simulink model "parrot_vision"  (R2020b)
settings: Solver=FixedStepAuto  StartTime=0.0  StopTime=100  RelTol=1e-3  EnableMultiTasking=on
InitFcn:
  | load('BusDefinitions.mat')
  | codertarget.parrot.internal.checkImageBlocks(gcs)
undefined symbols (not defined in the file): codertarget, Ts
libraries: simulink x3, parrotlib x1
settings Model: ExtModeTrigDuration=80  Creator=The MathWorks, Inc.  LastModifiedBy=anne
settings SolverCC: PositivePriorityOrder=on
settings DataIOCC: ReturnWorkspaceOutputs=off
settings OptimizationCC: PassReuseOutputArgsThreshold=0  MaxStackSize=64
settings DebuggingCC: ParameterTunabilityLossMsg=error  PregeneratedLibrarySubsystemCodeDiagnostic=none  ArithmeticOperatorsInVariantConditions=warning
settings HardwareCC: ProdBitPerPointer=32  ProdBitPerSizeT=32  ProdBitPerPtrDiffT=32  ProdLargestAtomicInteger=Long  ProdWordSize=32  ProdHWDeviceType=ARM Compatible->ARM 9  UseEmbeddedCoderFeatures=off  UseSimulinkCoderFeatures=off
settings SFSimCC: SimUseLocalCustomCode=off  MATLABDynamicMemAlloc=off  CustomCodeUndefinedFunction=UseInterfaceOnly
settings RTWCC: Description=Embedded Coder  SystemTargetFile=ert.tlc  HardwareBoard=PARROT Mambo  TemplateMakefile=ert_default_tmf  GenerateReport=on  RTWUseLocalCustomCode=off  Toolchain=Sourcery G++ Lite GNU Toolchain for Drones  LaunchReport=on
settings CodeAppCC: ForceParamTrailComments=on  OperatorAnnotations=on  StateflowObjectComments=on
settings ERTTargetCC: ERTCustomFileBanners=off  SupportContinuousTime=on  SupportNonInlinedSFcns=on  RemoveResetFunc=off  ModelStepFunctionPrototypeControlCompliant=off

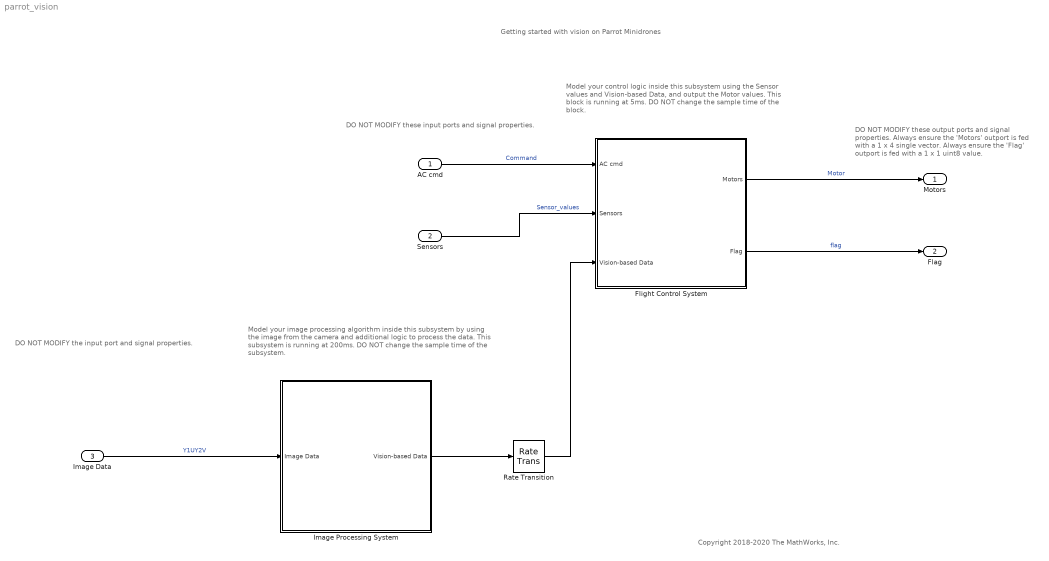
== system parrot_vision ==
  note: Model your control logic inside this subsystem
      | using the Sensor values and Vision-based Data,
      | and output the Motor values.
      | This block is running at 5ms.
      | DO NOT change the sample time of the block.
  note: DO NOT MODIFY these output ports
      | and signal properties.
      |
      |
      |
      |
      |
      | Always ensure the 'Motors' outport
      | is fed with a 1 x 4 single vector.
      |
      |
      |
      |
      |
      | Always ensure the 'Flag' outport is
      | fed with a 1 x 1 uint8 value.
  note: DO NOT MODIFY these input
      | ports and signal properties.
  note: Copyright 2018-2020 The MathWorks, Inc.
  note: Getting started with vision on Parrot Minidrones
  note: DO NOT MODIFY the input port and
      | signal properties.
  note: Model your image processing algorithm inside this
      | subsystem by using the image from the camera
      | and additional logic to process the data.
      | This subsystem is running at 200ms.
      | DO NOT change the sample time of the subsystem.
  AC cmd : Inport  OutDataTypeStr=Bus: CommandBus  BusOutputAsStruct=on
  Sensors : Inport  Port=2  OutDataTypeStr=Bus: SensorsBus  BusOutputAsStruct=on
  Image Data : Inport  Tag=IP_IN  InitFcn=codertarget.parrot.internal.inportCallback(gcb);  Port=3  OutDataTypeStr=uint8  PortDimensions=[4 9600]  BusOutputAsStruct=on
  Flight Control System : Subsystem  InitFcn=codertarget.parrot.internal.fcsSubsystemCallback(gcb);  TreatAsAtomicUnit=on  SystemSampleTime=Ts
  Image Processing System : Subsystem  Tag=IP_SUB  InitFcn=codertarget.parrot.internal.ipSubsystemCallback(gcb);  TreatAsAtomicUnit=on  SystemSampleTime=40*Ts  RTWFcnName=ImageFunction
      settings: RTWSystemCode=Inline  RTWFcnNameOpts=User specified
  Rate Transition : RateTransition  Deterministic=off
  Motors : Outport  OutDataTypeStr=single  PortDimensions=[1 4]  VectorParamsAs1DForOutWhenUnconnected=off
  Flag : Outport  Port=2  OutDataTypeStr=uint8  PortDimensions=1  VectorParamsAs1DForOutWhenUnconnected=off
  wires:
  Flight Control System/1(Motors) -> Motors/1  "Motor"
  AC cmd/1 -> Flight Control System/1(AC cmd)  "Command"
  Sensors/1 -> Flight Control System/2(Sensors)  "Sensor_values"
  Flight Control System/2(Flag) -> Flag/1  "flag"
  Image Data/1 -> Image Processing System/1(Image Data)  "Y1UY2V"
  Rate Transition/1 -> Flight Control System/3(" Vision-based Data")
  Image Processing System/1(" Vision-based Data") -> Rate Transition/1

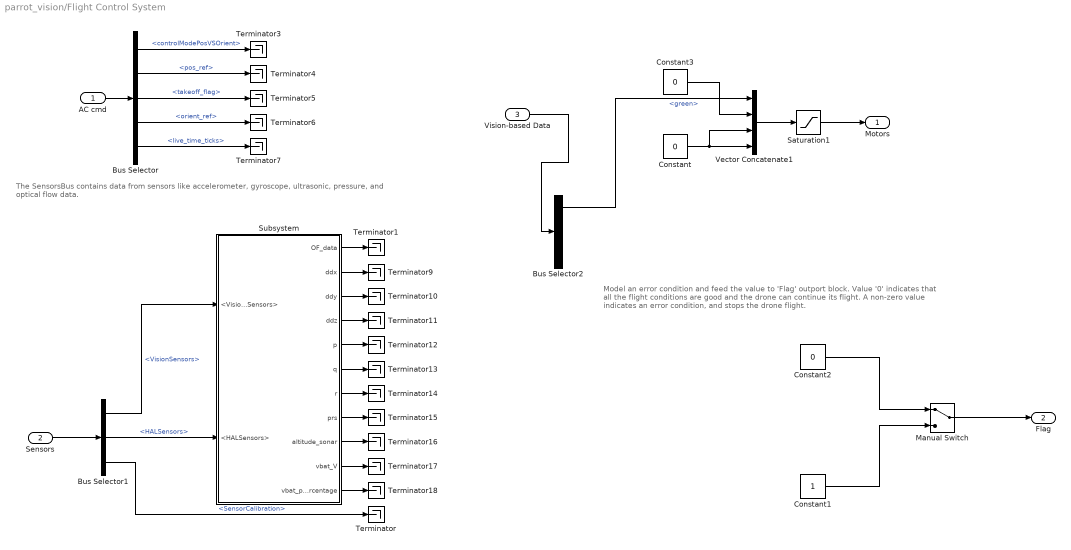
== system parrot_vision/Flight Control System ==
  note: Model an error condition and feed the value to 'Flag' outport block.
      | Value '0' indicates that all the flight conditions are good and the drone
      | can continue its flight.
      | A non-zero value indicates an error condition, and stops the drone
      | flight.
  note: The SensorsBus contains data from sensors like
      | accelerometer, gyroscope, ultrasonic, pressure,
      | and optical flow data.
  AC cmd : Inport
  Sensors : Inport  Port=2
  " Vision-based Data" : Inport  Port=3
  Bus Selector : BusSelector  OutputSignals=controlModePosVSOrient,pos_ref,takeoff_flag,orient_ref,live_time_ticks
  Bus Selector1 : BusSelector  OutputSignals=VisionSensors,HALSensors,SensorCalibration
  Bus Selector2 : BusSelector  OutputSignals=green,red,blue
  Constant : Constant  Value=0
  Constant1 : Constant  OutDataTypeStr=uint8
  Constant2 : Constant  Value=0  OutDataTypeStr=uint8
  Constant3 : Constant  Value=0
  Manual Switch : ManualSwitch
  Saturation1 : Saturate  UpperLimit=500  LowerLimit=0  OutDataTypeStr=single
  Subsystem : Subsystem
  Terminator{,1,3..7,9..18} (17 alike) : Terminator
  Vector Concatenate1 : Concatenate  NumInputs=4
  Motors : Outport  VectorParamsAs1DForOutWhenUnconnected=off
  Flag : Outport  Port=2  VectorParamsAs1DForOutWhenUnconnected=off
  wires:
  AC cmd/1 -> Bus Selector/1
  Sensors/1 -> Bus Selector1/1
  Bus Selector/1 -> Terminator3/1  "<controlModePosVSOrient>"
  Bus Selector/2 -> Terminator4/1  "<pos_ref>"
  Bus Selector/3 -> Terminator5/1  "<takeoff_flag>"
  Bus Selector/4 -> Terminator6/1  "<orient_ref>"
  Bus Selector/5 -> Terminator7/1  "<live_time_ticks>"
  Manual Switch/1 -> Flag/1
  Constant2/1 -> Manual Switch/1
  Constant1/1 -> Manual Switch/2
  Vector Concatenate1/1 -> Saturation1/1
  Saturation1/1 -> Motors/1
  Bus Selector1/1 -> Subsystem/1(<VisionSensors>)  "<VisionSensors>"
  Bus Selector1/2 -> Subsystem/2(<HALSensors>)  "<HALSensors>"
  Bus Selector1/3 -> Terminator/1  "<SensorCalibration>"
  Subsystem/1(OF_data) -> Terminator1/1
  Subsystem/2(ddx) -> Terminator9/1
  Subsystem/3(ddy) -> Terminator10/1
  Subsystem/4(ddz) -> Terminator11/1
  Subsystem/5(p) -> Terminator12/1
  Subsystem/7(r) -> Terminator14/1
  Subsystem/8(prs) -> Terminator15/1
  Subsystem/9(altitude_sonar) -> Terminator16/1
  Subsystem/10(vbat_V) -> Terminator17/1
  Subsystem/11(vbat_percentage) -> Terminator18/1
  Subsystem/6(q) -> Terminator13/1
  Constant/1 -> Vector Concatenate1/3, Vector Concatenate1/4
  " Vision-based Data"/1 -> Bus Selector2/1
  Bus Selector2/1 -> Vector Concatenate1/1  "<green>"
  Constant3/1 -> Vector Concatenate1/2

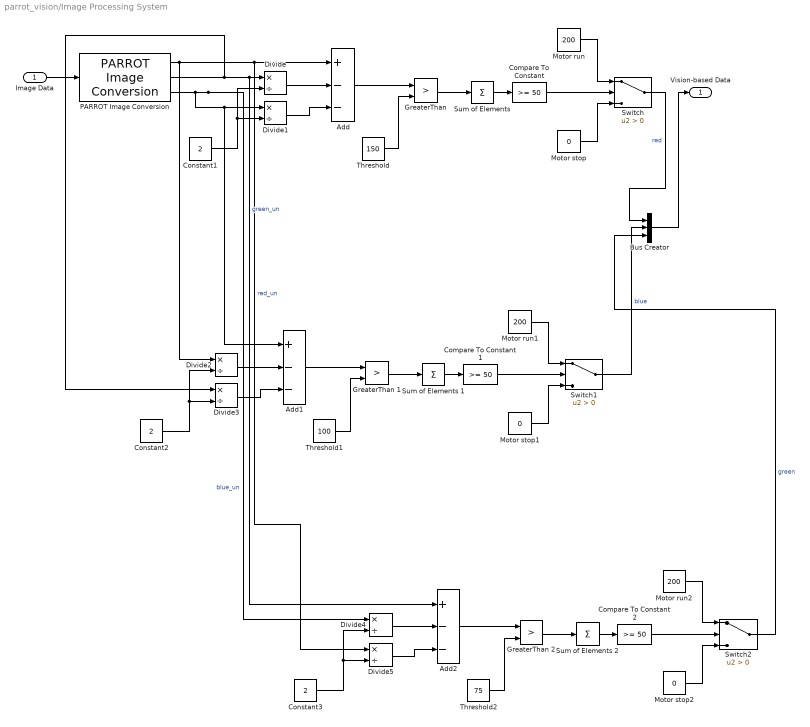
== system parrot_vision/Image Processing System ==
  Image Data : Inport
  Add : Sum  Inputs=+--
  Add1 : Sum  Inputs=+--
  Add2 : Sum  Inputs=+--
  Bus Creator : BusCreator  Inputs=3
  "Compare To Constant " : simulink/Logic and Bit Operations/Compare To Constant  relop=>=  const=50  OutDataTypeStr=boolean
  Compare To Constant 1 : simulink/Logic and Bit Operations/Compare To Constant  relop=>=  const=50  OutDataTypeStr=boolean
  Compare To Constant 2 : simulink/Logic and Bit Operations/Compare To Constant  relop=>=  const=50  OutDataTypeStr=boolean
  Constant1 : Constant  Value=2
  Constant2 : Constant  Value=2
  Constant3 : Constant  Value=2
  Divide{,1..5} (6 alike) : Product  Inputs=*/
  "GreaterThan " : RelationalOperator  Operator=>  OutDataTypeStr=boolean  RndMeth=Simplest
  GreaterThan 1 : RelationalOperator  Operator=>  OutDataTypeStr=boolean  RndMeth=Simplest
  GreaterThan 2 : RelationalOperator  Operator=>  OutDataTypeStr=boolean  RndMeth=Simplest
  Motor run : Constant  Value=200
  Motor run1 : Constant  Value=200
  Motor run2 : Constant  Value=200
  Motor stop : Constant  Value=0
  Motor stop1 : Constant  Value=0
  Motor stop2 : Constant  Value=0
  "PARROT Image Conversion " : parrotlib/PARROT Image Conversion  Tag=IP_FORMAT  ImageFormat=RGB  R=on  Y=on  G=on  U=on  B=on  V=on
      settings: SourceProductName=Simulink Support Package for Parrot Minidrones
  "Sum of Elements " : Sum  Inputs=+
  Sum of Elements 1 : Sum  Inputs=+
  Sum of Elements 2 : Sum  Inputs=+
  Switch : Switch  Criteria=u2 > Threshold
  Switch1 : Switch  Criteria=u2 > Threshold
  Switch2 : Switch  Criteria=u2 > Threshold
  Threshold : Constant  Value=150
  Threshold1 : Constant  Value=100
  Threshold2 : Constant  Value=75
  " Vision-based Data" : Outport  VectorParamsAs1DForOutWhenUnconnected=off
  wires:
  Divide1/1 -> Add/3
  "Sum of Elements "/1 -> "Compare To Constant "/1
  "Compare To Constant "/1 -> Switch/2
  Image Data/1 -> "PARROT Image Conversion "/1
  Threshold/1 -> "GreaterThan "/2
  Motor run/1 -> Switch/1
  Constant1/1 -> Divide1/2, Divide/2
  Add/1 -> "GreaterThan "/1
  "GreaterThan "/1 -> "Sum of Elements "/1
  Divide/1 -> Add/2
  Motor stop/1 -> Switch/3
  Constant2/1 -> Divide3/2, Divide2/2
  Add1/1 -> GreaterThan 1/1
  Divide2/1 -> Add1/2
  Divide3/1 -> Add1/3
  Motor run1/1 -> Switch1/1
  Threshold1/1 -> GreaterThan 1/2
  Compare To Constant 1/1 -> Switch1/2
  GreaterThan 1/1 -> Sum of Elements 1/1
  Sum of Elements 1/1 -> Compare To Constant 1/1
  Motor stop1/1 -> Switch1/3
  Bus Creator/1 -> " Vision-based Data"/1
  Switch1/1 -> Bus Creator/2  "blue"
  Constant3/1 -> Divide5/2, Divide4/2
  Add2/1 -> GreaterThan 2/1
  Divide4/1 -> Add2/2
  Divide5/1 -> Add2/3
  "PARROT Image Conversion "/1 -> Divide5/1, Add/1, Divide2/1  "red_un"
  Motor run2/1 -> Switch2/1
  Threshold2/1 -> GreaterThan 2/2
  Compare To Constant 2/1 -> Switch2/2
  GreaterThan 2/1 -> Sum of Elements 2/1
  Sum of Elements 2/1 -> Compare To Constant 2/1
  "PARROT Image Conversion "/2 -> Add2/1, Divide/1, Divide3/1  "green_un"
  "PARROT Image Conversion "/3 -> Divide4/1, Add1/1, Divide1/1  "blue_un"
  Motor stop2/1 -> Switch2/3
  Switch2/1 -> Bus Creator/3  "green"
  Switch/1 -> Bus Creator/1  "red"

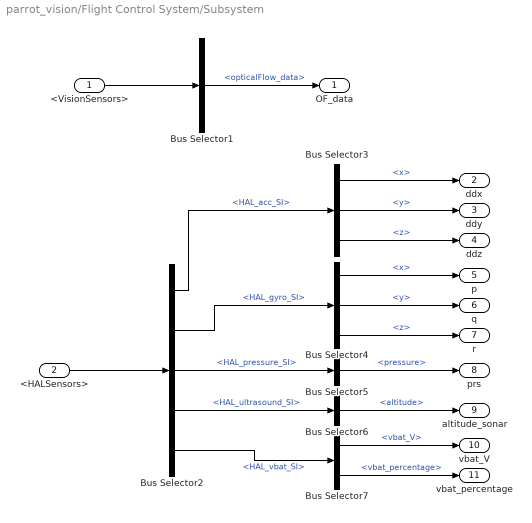
== system parrot_vision/Flight Control System/Subsystem ==
  <VisionSensors> : Inport
  <HALSensors> : Inport  Port=2
  Bus Selector1 : BusSelector  OutputSignals=opticalFlow_data
  Bus Selector2 : BusSelector  OutputSignals=HAL_acc_SI,HAL_gyro_SI,HAL_pressure_SI,HAL_ultrasound_SI,HAL_vbat_SI
  Bus Selector3 : BusSelector  OutputSignals=x,y,z
  Bus Selector4 : BusSelector  OutputSignals=x,y,z
  Bus Selector5 : BusSelector  OutputSignals=pressure
  Bus Selector6 : BusSelector  OutputSignals=altitude
  Bus Selector7 : BusSelector  OutputSignals=vbat_V,vbat_percentage
  OF_data : Outport  VectorParamsAs1DForOutWhenUnconnected=off
  ddx : Outport  Port=2  VectorParamsAs1DForOutWhenUnconnected=off
  ddy : Outport  Port=3  VectorParamsAs1DForOutWhenUnconnected=off
  ddz : Outport  Port=4  VectorParamsAs1DForOutWhenUnconnected=off
  p : Outport  Port=5  VectorParamsAs1DForOutWhenUnconnected=off
  q : Outport  Port=6  VectorParamsAs1DForOutWhenUnconnected=off
  r : Outport  Port=7  VectorParamsAs1DForOutWhenUnconnected=off
  prs : Outport  Port=8  VectorParamsAs1DForOutWhenUnconnected=off
  altitude_sonar : Outport  Port=9  VectorParamsAs1DForOutWhenUnconnected=off
  vbat_V : Outport  Port=10  VectorParamsAs1DForOutWhenUnconnected=off
  vbat_percentage : Outport  Port=11  VectorParamsAs1DForOutWhenUnconnected=off
  wires:
  <VisionSensors>/1 -> Bus Selector1/1
  <HALSensors>/1 -> Bus Selector2/1
  Bus Selector1/1 -> OF_data/1  "<opticalFlow_data>"
  Bus Selector2/1 -> Bus Selector3/1  "<HAL_acc_SI>"
  Bus Selector2/2 -> Bus Selector4/1  "<HAL_gyro_SI>"
  Bus Selector2/3 -> Bus Selector5/1  "<HAL_pressure_SI>"
  Bus Selector2/4 -> Bus Selector6/1  "<HAL_ultrasound_SI>"
  Bus Selector2/5 -> Bus Selector7/1  "<HAL_vbat_SI>"
  Bus Selector3/1 -> ddx/1  "<x>"
  Bus Selector3/2 -> ddy/1  "<y>"
  Bus Selector3/3 -> ddz/1  "<z>"
  Bus Selector4/2 -> q/1  "<y>"
  Bus Selector4/1 -> p/1  "<x>"
  Bus Selector4/3 -> r/1  "<z>"
  Bus Selector5/1 -> prs/1  "<pressure>"
  Bus Selector6/1 -> altitude_sonar/1  "<altitude>"
  Bus Selector7/1 -> vbat_V/1  "<vbat_V>"
  Bus Selector7/2 -> vbat_percentage/1  "<vbat_percentage>"
